simulink model "LQR_pade_observer_discrete"  (R2023b)
settings: Solver=VariableStepAuto  StartTime=0.0  StopTime=20  FixedStep=Ts  RelTol=1e-3
values from neighbouring files (symbols this model uses):
  A = sys_pade.A    [attempt.m]    (also in model_approximation.m; observer.m = [-7.9641 0 8.7857; 1.0000 0 0; 0 0 -35.1427]; progetto.m = [0 1; 0 -1/Tm]; tuning.m)
  B = sys_pade.B    [attempt.m]    (also in model_approximation.m; observer.m = [-1;0;8]; progetto.m = [0 ;km/Tm]; tuning.m)
  C = sys_pade.C    [attempt.m]    (also in model_approximation.m; observer.m = [0, 5.6163, 0]; progetto.m = [1 0]; tuning.m)
  K_tilde = [1.0706    9.0642    0.2639   -0.7581]    [observer.m]
  kr = -1/(C*inv(A-B*K_tilde(1:3))*B)    [controller_tuning.m]    (also in observer.m; progetto.m = -1/(C*inv(A-B*K)*B); tuning.m)
  L = [l1;l2;l3]    [observer.m]    (also in torque.m = 0.0082)
  r = 50    [progetto.m]
  sys_discrete = c2d(sys_continuos,0.005,'tustin')    [observer.m]
  Ts = 0.005    [attempt.m]    (also in model_approximation.m; tuning.m)
undefined symbols (not defined in the file or in its folder): disturbance
settings Model: Creator=giova  LastModifiedBy=giova

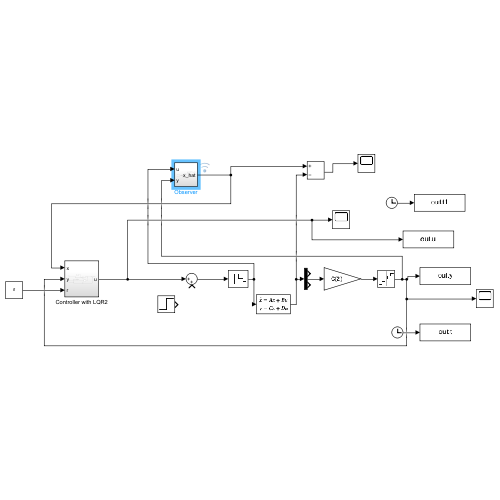
[thumbnail: Simulink's stored preview of the top-level diagram]
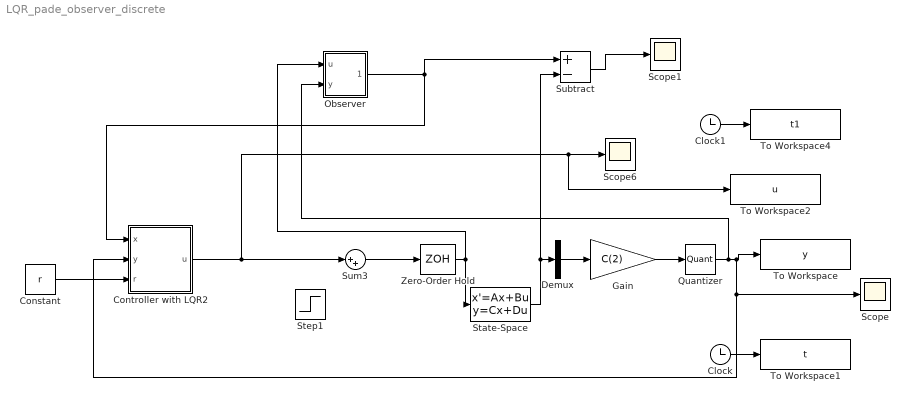
== system LQR_pade_observer_discrete ==
  Clock : Clock
  Clock1 : Clock
  Constant : Constant  Value=r
  Controller with LQR2 : Subsystem
  Demux : Demux  Outputs=3
  Gain : Gain  Gain=C(2)
  Observer : Subsystem
  Quantizer : Quantizer  QuantizationInterval=Ts
  Scope : Scope
  Scope1 : Scope
  Scope6 : Scope
  State-Space : StateSpace  A=A  B=B  C=eye(3)  D=[0;0;0]  InitialCondition=0
  Step1 : Step  Time=2  After=disturbance  SampleTime=0
  Subtract : Sum  Inputs=+-
  Sum3 : Sum  Inputs=|++
  To Workspace : ToWorkspace  VariableName=y  SampleTime=-1
  To Workspace1 : ToWorkspace  VariableName=t  SampleTime=-1
  To Workspace2 : ToWorkspace  VariableName=u  SampleTime=-1
  To Workspace4 : ToWorkspace  VariableName=t1  SampleTime=-1
  Zero-Order Hold : ZeroOrderHold  SampleTime=Ts
  wires:
  Sum3/1 -> Zero-Order Hold/1
  Controller with LQR2/1(u) -> To Workspace2/1, Scope6/1, Sum3/1
  Clock/1 -> To Workspace1/1
  Clock1/1 -> To Workspace4/1
  Constant/1 -> Controller with LQR2/3(r)
  Observer/1(x_hat) -> Controller with LQR2/1(x), Subtract/1
  Demux/2 -> Gain/1
  Subtract/1 -> Scope1/1
  Gain/1 -> Quantizer/1
  Quantizer/1 -> Observer/2(y), Controller with LQR2/2(y), Scope/1, To Workspace/1
  State-Space/1 -> Subtract/2, Demux/1
  Zero-Order Hold/1 -> Observer/1(u), State-Space/1

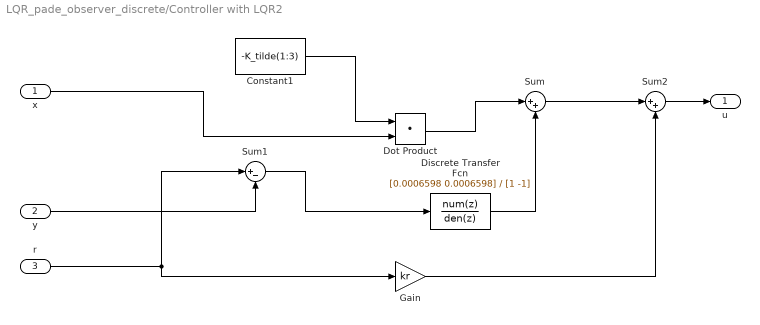
== system LQR_pade_observer_discrete/Controller with LQR2 ==
  x : Inport
  y : Inport  Port=2
  r : Inport  Port=3
  Constant1 : Constant  Value=-K_tilde(1:3)
  Discrete Transfer Fcn : DiscreteTransferFcn  Numerator=[0.0006598 0.0006598]  Denominator=[1 -1]  SampleTime=Ts  StateName='slowIntState'
  Dot Product : DotProduct  OutDataTypeStr=Inherit: Inherit via internal rule
  Gain : Gain  Gain=kr
  Sum : Sum  Inputs=|++
  Sum1 : Sum  Inputs=|+-
  Sum2 : Sum  Inputs=|++
  u : Outport
  wires:
  Dot Product/1 -> Sum/1
  Discrete Transfer Fcn/1 -> Sum/2
  Sum1/1 -> Discrete Transfer Fcn/1
  y/1 -> Sum1/2
  x/1 -> Dot Product/2
  Sum2/1 -> u/1
  Constant1/1 -> Dot Product/1
  Gain/1 -> Sum2/2
  Sum/1 -> Sum2/1
  r/1 -> Gain/1, Sum1/1

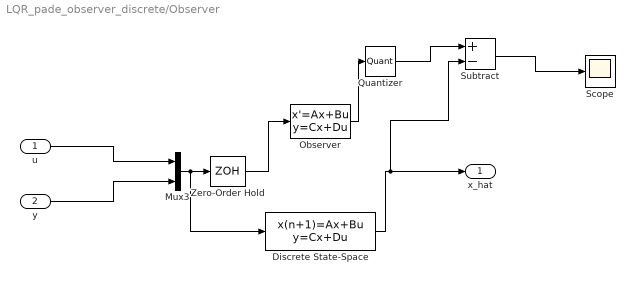
== system LQR_pade_observer_discrete/Observer ==
  u : Inport
  y : Inport  Port=2
  Discrete State-Space : DiscreteStateSpace  A=sys_discrete.A  B=sys_discrete.B  C=sys_discrete.C  D=sys_discrete.D  SampleTime=Ts
  Mux3 : Mux  Inputs=2
  Observer : StateSpace  A=A-L*C  B=[B L]  C=eye(3)  D=[0 0; 0 0; 0 0]  InitialCondition=[0 0 0]  ParameterTunability=Unconstrained
  Quantizer : Quantizer  QuantizationInterval=Ts
  Scope : Scope
  Subtract : Sum  Inputs=+-
  Zero-Order Hold : ZeroOrderHold  SampleTime=-1
  x_hat : Outport
  wires:
  y/1 -> Mux3/2
  u/1 -> Mux3/1
  Mux3/1 -> Discrete State-Space/1, Zero-Order Hold/1
  Zero-Order Hold/1 -> Observer/1
  Discrete State-Space/1 -> Subtract/2, x_hat/1
  Observer/1 -> Quantizer/1
  Quantizer/1 -> Subtract/1
  Subtract/1 -> Scope/1
